simulink model "FILTRO"  (R2014a)
settings: Solver=ode45  StartTime=0.0  StopTime=0.000655  RelTol=1e-3
values from neighbouring files (symbols this model uses):
  SampleTime = 3.25520833333e-06    [sigma-delta.mat]
libraries: dspsigops x2
settings Model: Creator=FaNar  LastModifiedBy=root

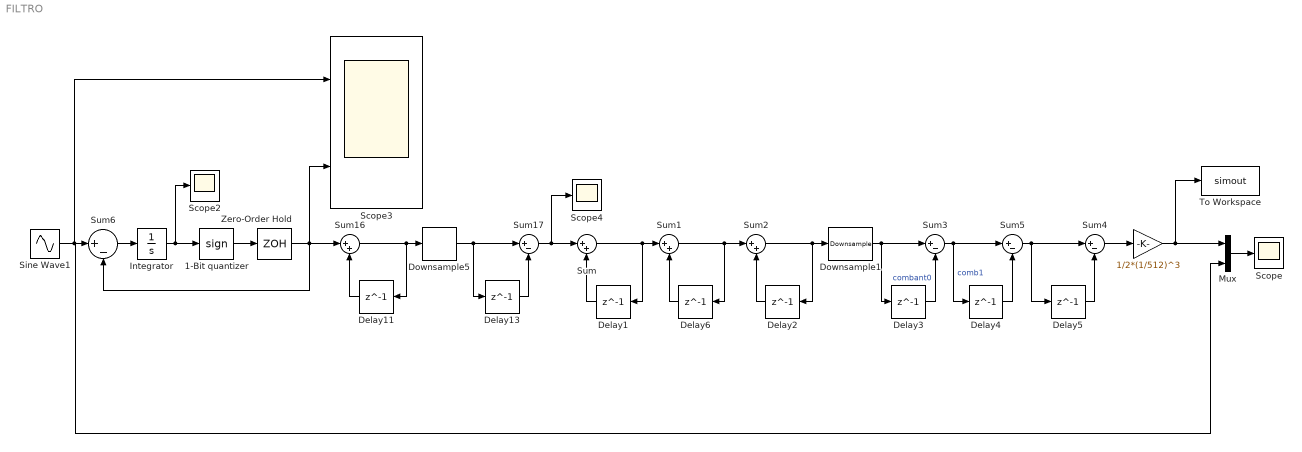
== system FILTRO ==
  " " : Gain  Gain=1/2*(1/512)^3
  1-Bit quantizer : Signum
  Delay{1..6,11,13} (8 alike) : Delay  DelayLength=1
  Downsample1 : dspsigops/Downsample  N=512  phase=0  RateOptions=Allow multirate processing  smode=Allow multirate  fmode=Maintain input frame size  ic=0
  Downsample5 : dspsigops/Downsample  N=2  phase=0  RateOptions=Allow multirate processing  smode=Allow multirate  fmode=Maintain input frame size  ic=0
  Integrator : Integrator
  Mux : Mux  Inputs=2
  Scope : Scope
      settings: TimeRange=0.001  YMin=-0.9  YMax=1
  Scope2 : Scope
      settings: TimeRange=0.0003  YMin=2.5e-05  YMax=0.000275  SaveName=ScopeData2
  Scope3 : Scope  NumInputPorts=2
      settings: TimeRange=0.0002  YMin=-11000~0.95  YMax=11000~1.05  SaveName=ScopeData3
  Scope4 : Scope
      settings: TimeRange=100  YMin=0.95  YMax=1.05  SaveName=ScopeData4
  Sine Wave1 : Sin  Frequency=50000*2*pi  SampleTime=0
  Sum{,1..2,16} (4 alike) : Sum  Inputs=|++
  Sum{3..5,17} (4 alike) : Sum  Inputs=|+-
  Sum6 : Sum  Inputs=|+-  SaturateOnIntegerOverflow=on  InputSameDT=on  OutDataTypeStr=Inherit: Same as first input
  To Workspace : ToWorkspace  VariableName=simout  SampleTime=-1
      settings: Save2DSignal=2-D array (concatenate along first dimension)
  Zero-Order Hold : ZeroOrderHold  SampleTime=SampleTime
  wires:
  Delay1/1 -> Sum/2
  Sum/1 -> Sum1/1, Delay1/1
  Delay4/1 -> Sum5/2
  Delay6/1 -> Sum1/2
  Sum1/1 -> Sum2/1, Delay6/1
  Delay2/1 -> Sum2/2
  Delay3/1 -> Sum3/2  "combant0"
  Sum3/1 -> Sum5/1, Delay4/1  "comb1"
  Delay5/1 -> Sum4/2
  Sum5/1 -> Sum4/1, Delay5/1
  Sine Wave1/1 -> Scope3/1, Mux/2, Sum6/1
  Zero-Order Hold/1 -> Sum6/2, Sum16/1, Scope3/2
  1-Bit quantizer/1 -> Zero-Order Hold/1
  Sum6/1 -> Integrator/1
  Integrator/1 -> 1-Bit quantizer/1, Scope2/1
  Sum2/1 -> Downsample1/1, Delay2/1
  Delay11/1 -> Sum16/2
  Sum16/1 -> Delay11/1, Downsample5/1
  Delay13/1 -> Sum17/2
  Downsample5/1 -> Sum17/1, Delay13/1
  Downsample1/1 -> Delay3/1, Sum3/1
  Sum4/1 -> " "/1
  Mux/1 -> Scope/1
  " "/1 -> Mux/1, To Workspace/1
  Sum17/1 -> Sum/1, Scope4/1
